simulink model "sim_ecualizador"  (R2020b)
settings: Solver=VariableStepAuto  StartTime=0.0  StopTime=inf  RelTol=1e-3
libraries: dsparch4 x6, dspmathops x6, dspsnks4 x1, dspvision x1
settings Model: Creator=Daniel Ramírez  LastModifiedBy=Daniel Ramírez

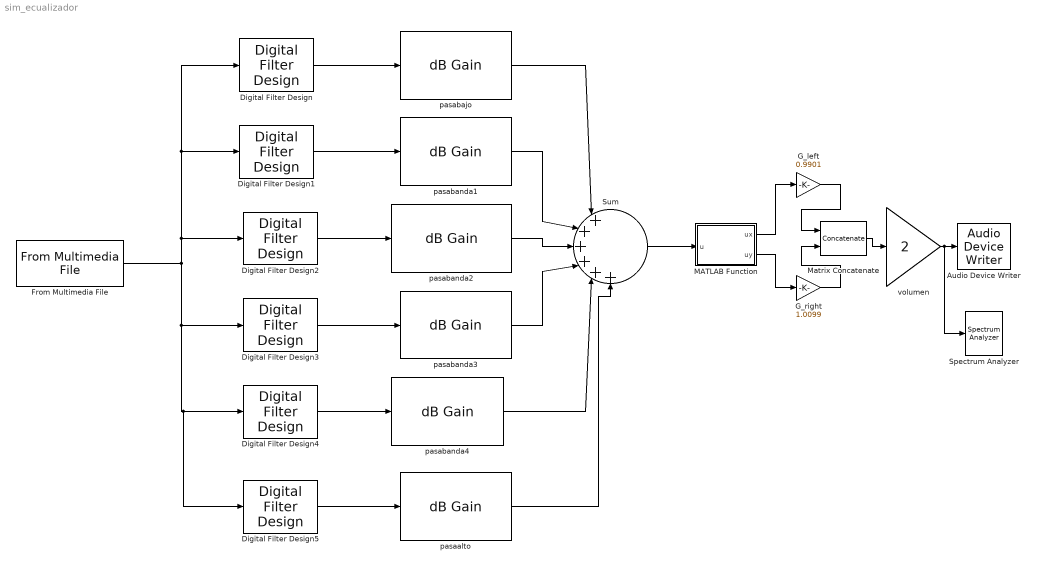
== system sim_ecualizador ==
  Audio Device Writer : dspsnks4/Audio Device Writer  Driver=DirectSound  Device=Default  InheritSampleRate=on  SampleRate=44100  BitDepth=16-bit integer  BufferSize=4096  NumBuffers=10  DefaultOutputChannelMapping=on  OutputChannelMapping=1:2  OutputNumUnderrunSamples=off  DriverIdx=1  DeviceWarnFlag=''
  Digital Filter Design{,1..5} (6 alike) : dsparch4/Digital Filter Design  mwdsp_browser_bugfix_var=off
  From Multimedia File : dspvision/From Multimedia File  inputFilename=C:\Users\Daniel Ramírez\OneDrive\Escritorio\cod_matlab2021\audio_sim.wav  readRange=[1 Inf]  loop=on  numPlays=inf  outputStreams=Audio only  videoDataType=single  audioDataType=double  inheritSampleTime=on  userDefinedSampleTime=1/30  noAudioOutput=off  isIntensityVideo=off  fourcc=RGB  colorVideoFormat=Separate color signals  outputEOF=off  dataOrg=Column-major  audioFrameSize=1024  computeAudioFrameSize=off  outSamplingMode=Sample based
  G_left : Gain  Gain=0.9901
  G_right : Gain  Gain=1.0099
  MATLAB Function : MATLAB Function  TreatAsAtomicUnit=on
  Matrix Concatenate : Concatenate  Mode=Multidimensional array  ConcatenateDimension=2
  Spectrum Analyzer : SpectrumAnalyzer
  Sum : Sum  Inputs=|++++++
  pasaalto : dspmathops/dB Gain  dB=0.5  intype=Amplitude
      settings: SourceProductBaseCode=DS
  pasabajo : dspmathops/dB Gain  dB=-15  intype=Amplitude
      settings: SourceProductBaseCode=DS
  pasabanda1 : dspmathops/dB Gain  dB=-6.8317  intype=Amplitude
      settings: SourceProductBaseCode=DS
  pasabanda2 : dspmathops/dB Gain  dB=-9.802  intype=Amplitude
      settings: SourceProductBaseCode=DS
  pasabanda3 : dspmathops/dB Gain  dB=8.4653  intype=Amplitude
      settings: SourceProductBaseCode=DS
  pasabanda4 : dspmathops/dB Gain  dB=-0.89109  intype=Amplitude
      settings: SourceProductBaseCode=DS
  volumen : Gain  Gain=2
  wires:
  Digital Filter Design5/1 -> pasaalto/1
  Digital Filter Design4/1 -> pasabanda4/1
  Digital Filter Design3/1 -> pasabanda3/1
  Digital Filter Design2/1 -> pasabanda2/1
  Digital Filter Design1/1 -> pasabanda1/1
  Digital Filter Design/1 -> pasabajo/1
  From Multimedia File/1 -> Digital Filter Design5/1, Digital Filter Design4/1, Digital Filter Design3/1, Digital Filter Design2/1, Digital Filter Design1/1, Digital Filter Design/1
  pasabajo/1 -> Sum/1
  pasabanda1/1 -> Sum/2
  pasabanda2/1 -> Sum/3
  pasabanda3/1 -> Sum/4
  pasabanda4/1 -> Sum/5
  pasaalto/1 -> Sum/6
  volumen/1 -> Spectrum Analyzer/1, Audio Device Writer/1
  Sum/1 -> MATLAB Function/1(u)
  MATLAB Function/1(ux) -> G_left/1
  MATLAB Function/2(uy) -> G_right/1
  G_left/1 -> Matrix Concatenate/1
  G_right/1 -> Matrix Concatenate/2
  Matrix Concatenate/1 -> volumen/1

== matlab function sim_ecualizador/MATLAB Function ==
  data: u input; ux output; uy output
function [ux,uy] = fcn(u)

ux = u(:,1);
uy = u(:,2);
